simulink model "first"  (R2024a)
settings: Solver=VariableStepAuto  StartTime=0.0  StopTime=2  RelTol=1e-3
values from neighbouring files (symbols this model uses):
  K_CO = 7.2    [first_calc.m]
  K_FB = -1    [first_calc.m]
  T = 0.2    [first_calc.m]    (also in second.m; third_calc.m = 0.25)
settings Model: Creator=ventus  LastModifiedBy=ventus

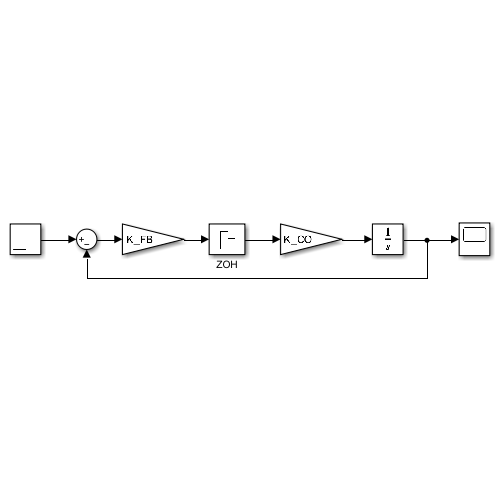
[thumbnail: Simulink's stored preview of the top-level diagram]
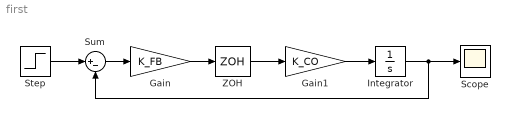
== system first ==
  Gain : Gain  Gain=K_FB
  Gain1 : Gain  Gain=K_CO
  Integrator : Integrator
  Scope : Scope
  Step : Step  SampleTime=0
  Sum : Sum  Inputs=|+-
  ZOH : ZeroOrderHold  SampleTime=T
  wires:
  Step/1 -> Sum/1
  Sum/1 -> Gain/1
  Gain/1 -> ZOH/1
  ZOH/1 -> Gain1/1
  Gain1/1 -> Integrator/1
  Integrator/1 -> Sum/2, Scope/1
